simulink model "FreqAdaptive"  (R2018a)
settings: Solver=ode8  StartTime=0.0  StopTime=Ttot  FixedStep=Ts  RelTol=1e-3
values from neighbouring files (symbols this model uses):
  Fn = 60    [Equivalency_Script.m]    (also in FreqAdaptiveFFT_Script.m; FreqAdaptive_Script.m; ShortPulse_Script.m)
  Ts = Ts_control / 60    (= 9.25925925926e-07)    [Equivalency_Script.m]    (also in FreqAdaptiveFFT_Script.m; FreqAdaptive_Script.m; ShortPulse_Script.m)
  Ts_control = 1/(300*Fn)    (= 5.55555555556e-05)    [Equivalency_Script.m]    (also in FreqAdaptiveFFT_Script.m; FreqAdaptive_Script.m; ShortPulse_Script.m)
libraries: powerlib x3, DSCdq_Library x2, powerlib_meascontrol x2
settings Model: SimulationMode=accelerator  Creator=daniemot  LastModifiedBy=daniemot
settings SolverCC: AutoInsertRateTranBlk=on
settings DataIOCC: ExternalInput=getinputstruct(WN_50mF_op_snapshot1)  InitialState=getstatestruct(WN_50mF_op_snapshot1)  SaveFinalState=on  SaveFormat=StructureWithTime  SaveOutput=off  SignalLogging=off  DSMLogging=off  SaveTime=off
settings DebuggingCC: ReadBeforeWriteMsg=DisableAll  WriteAfterWriteMsg=DisableAll  WriteAfterReadMsg=DisableAll  MultiTaskDSMMsg=none  UnconnectedInputMsg=none  UnconnectedOutputMsg=none  UnconnectedLineMsg=none
settings ModelReferenceCC: UpdateModelReferenceTargets=IfOutOfDate
settings SFSimCC: SFSimEcho=off

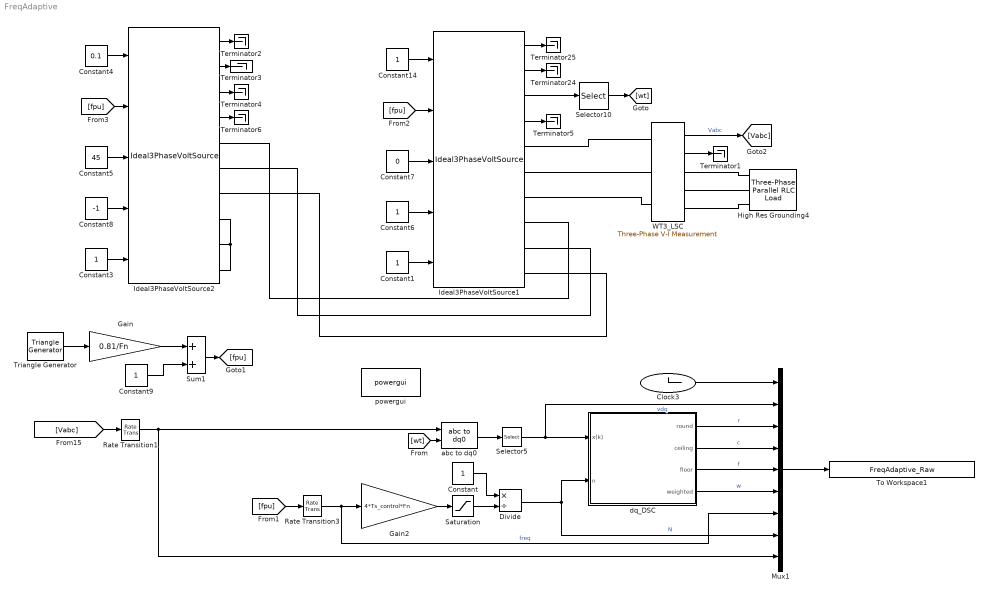
== system FreqAdaptive ==
  Clock3 : Clock
  Constant{,1,3,6,9,14} (6 alike) : Constant
  Constant4 : Constant  Value=0.1
  Constant5 : Constant  Value=45
  Constant7 : Constant  Value=0
  Constant8 : Constant  Value=-1
  Divide : Product  Inputs=*/
  Gain : Gain  Gain=0.81/Fn
  Gain2 : Gain  Gain=4*Ts_control*Fn
  High Res Grounding4 : powerlib/Elements/Three-Phase Parallel RLC Load  LConnTagsString=A|B|C  Configuration=Y (grounded)  NominalVoltage=(1/2^0.5)*3^0.5  Vabc=[1e3 1e3 1e3]  Vabcp=[1e3 1e3 1e3]  NominalFrequency=Fn  UnbalancedPower=off  ActivePower=3/2  InductivePower=0  CapacitivePower=0  Pabc=[10e3 9e3 11e3]  QLabc=[100 90 110]  QCabc=[100 90 110]  Pabcp=[10e3 9e3 11e3]  QLabcp=[100 90 110]  QCabcp=[100 90 110]  Measurements=None  LoadType=constant Z
  Ideal3PhaseVoltSource1 : DSCdq_Library/Ideal3PhaseVoltSource  BaseAmp=1  fn=Fn
  Ideal3PhaseVoltSource2 : DSCdq_Library/Ideal3PhaseVoltSource  BaseAmp=1  fn=Fn
  Mux1 : Mux  Inputs=9
  Rate Transition1 : RateTransition  OutPortSampleTime=Ts_control
  Rate Transition3 : RateTransition  InitialCondition=1  OutPortSampleTime=Ts_control
  Saturation : Saturate  UpperLimit=inf  LowerLimit=0.000001
  Selector10 : Selector  InputPortWidth=3  IndexOptions=Index vector (dialog)  Indices=[1]  OutputSizes=1
  Selector5 : Selector  InputPortWidth=3  IndexOptions=Index vector (dialog)  Indices=[1 2]  OutputSizes=1
  Sum1 : Sum
  Terminator{1..6,24..25} (8 alike) : Terminator
  To Workspace1 : ToWorkspace  VariableName=FreqAdaptive_Raw  SampleTime=Ts_control
      settings: Save2DSignal=2-D array (concatenate along first dimension)
  Triangle Generator : powerlib_meascontrol/Pulse & Signal Generators/Triangle Generator  Freq=2  Phase=90  Ts=0
  WT3_LSC : powerlib/Measurements/Three-Phase V-I Measurement  VoltageMeasurement=phase-to-ground  SetLabelV=off  LabelV=vgrid  Vpu=off  VpuLL=off  CurrentMeasurement=yes  SetLabelI=off  LabelI=igrid  Ipu=off  Pbase=sn  Vbase=uab  OutputType=Complex  PhasorSimulation=off  PSBequivalent=0
  abc to dq0 : powerlib_meascontrol/Transformations/abc to dq0  Alignment=90 degrees behind phase A axis
  dq_DSC : Subsystem  TreatAsAtomicUnit=on  SystemSampleTime=Ts  mask{Ts=Ts_control, nmax=200}
      mask prompts: Ts "Sample times [s]"; nmax "Maximum delay nmax:"
      mask Display: fprintf('y(k)=0.5(x(k)+x(k-n))');
  powergui : powerlib/powergui  Priority=1  SimulationMode=Discrete  SampleTime=Ts  frequency=60  Iterations=50  frequencyindice=0  Pbase=100e6  ErrMax=1e-4  UnitsV=kV  UnitsW=MW  buscounter=0  FunctionMessages=off  echomessages=off  EnableUseOfTLC=off  CurrentSourceSwitches=off  DisableSnubberDevices=off  DisableRonSwitches=off  DisableVfSwitches=off  DisplayEquations=off  SolverType=Tustin/Backward Euler (TBE)  Interpol=off  ExternalGateDelay=off  methode=off  Ts=100  x0status=blocks  SPID=off  SwTol=0  HookPort=off  RestoreLinks=warning  ResistiveCurrentMeasurement=off  Frange=[60:1:1600]  Ylog=on  Xlog=on  ShowGrid=on  save=off  variable=ZData  structure=0  ZoomFFT=off  StartTime=0.0  cycles=1  DisplayStyle=1  fundamental=60  FreqAxis=off  MaxFrequency=1000  frequencyindicesteady=1  RmsSteady=1  display=off
  wires:
  Constant6/1 -> Ideal3PhaseVoltSource1/4
  Constant7/1 -> Ideal3PhaseVoltSource1/3
  Triangle Generator/1 -> Gain/1
  Ideal3PhaseVoltSource1/3 -> Selector10/1
  Ideal3PhaseVoltSource1/2 -> Terminator24/1
  Ideal3PhaseVoltSource1/1 -> Terminator25/1
  WT3_LSC/1 -> [Vabc]  "Vabc"
  Ideal3PhaseVoltSource1/4 -> Terminator5/1
  Clock3/1 -> Mux1/1
  Mux1/1 -> To Workspace1/1
  Constant14/1 -> Ideal3PhaseVoltSource1/1
  Constant1/1 -> Ideal3PhaseVoltSource1/5
  WT3_LSC/2 -> Terminator1/1
  Selector5/1 -> Mux1/2, dq_DSC/1(x(k))  "vdq"
  [wt] -> abc to dq0/2
  abc to dq0/1 -> Selector5/1
  [Vabc] -> Rate Transition1/1
  Divide/1 -> Mux1/8, dq_DSC/2(n)  "N"
  Constant/1 -> Divide/1
  [fpu] -> Rate Transition3/1
  Gain2/1 -> Saturation/1
  Saturation/1 -> Divide/2
  dq_DSC/1(round) -> Mux1/3  "r"
  dq_DSC/2(ceiling) -> Mux1/4  "c"
  dq_DSC/3(floor) -> Mux1/5  "f"
  dq_DSC/4(weighted) -> Mux1/6  "w"
  Rate Transition3/1 -> Mux1/7, Gain2/1  "freq"
  Ideal3PhaseVoltSource2/1 -> Terminator2/1
  Ideal3PhaseVoltSource2/2 -> Terminator3/1
  Ideal3PhaseVoltSource2/3 -> Terminator4/1
  Ideal3PhaseVoltSource2/4 -> Terminator6/1
  Constant3/1 -> Ideal3PhaseVoltSource2/5
  [fpu] -> Ideal3PhaseVoltSource2/2
  Constant4/1 -> Ideal3PhaseVoltSource2/1
  Constant5/1 -> Ideal3PhaseVoltSource2/3
  Constant8/1 -> Ideal3PhaseVoltSource2/4
  Sum1/1 -> [fpu]
  Gain/1 -> Sum1/1
  Constant9/1 -> Sum1/2
  Rate Transition1/1 -> abc to dq0/1, Mux1/9
  [fpu] -> Ideal3PhaseVoltSource1/2
  Selector10/1 -> [wt]
  connections:
  Ideal3PhaseVoltSource1/RConn1 -- WT3_LSC/LConn1
  Ideal3PhaseVoltSource1/RConn3 -- WT3_LSC/LConn3
  Ideal3PhaseVoltSource1/RConn2 -- WT3_LSC/LConn2
  High Res Grounding4/LConn1 -- WT3_LSC/RConn1
  High Res Grounding4/LConn2 -- WT3_LSC/RConn2
  High Res Grounding4/LConn3 -- WT3_LSC/RConn3
  Ideal3PhaseVoltSource2/RConn4 -- Ideal3PhaseVoltSource2/RConn6 -- Ideal3PhaseVoltSource2/RConn5
  Ideal3PhaseVoltSource1/RConn6 -- Ideal3PhaseVoltSource2/RConn3
  Ideal3PhaseVoltSource1/RConn5 -- Ideal3PhaseVoltSource2/RConn2
  Ideal3PhaseVoltSource1/RConn4 -- Ideal3PhaseVoltSource2/RConn1

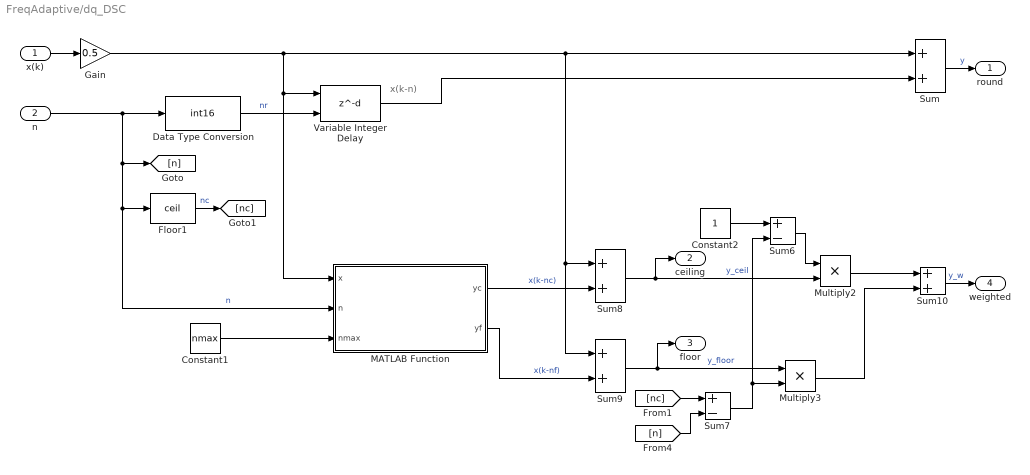
== system FreqAdaptive/dq_DSC ==
  note: x(k-n)
  x(k) : Inport
  n : Inport  Port=2
  Constant1 : Constant  Value=nmax
  Constant2 : Constant
  Data Type Conversion : DataTypeConversion  OutDataTypeStr=int16  RndMeth=Round  SaturateOnIntegerOverflow=on
  Floor1 : Rounding  Operator=ceil
  Gain : Gain  Gain=0.5
  MATLAB Function : MATLAB Function  TreatAsAtomicUnit=on  SystemSampleTime=Ts_control
  Multiply2 : Product
  Multiply3 : Product
  Sum{,8..10} (4 alike) : Sum
  Sum6 : Sum  Inputs=+-
  Sum7 : Sum  Inputs=+-
  Variable Integer Delay : Delay  DelayLengthSource=Input port  DelayLength=200  DelayLengthUpperLimit=nmax  SampleTime=Ts
      settings: InputPortMap=u0,p1
  round : Outport
  ceiling : Outport  Port=2
  floor : Outport  Port=3
  weighted : Outport  Port=4
  wires:
  Sum/1 -> round/1  "y"
  Data Type Conversion/1 -> Variable Integer Delay/2  "nr"
  Floor1/1 -> [nc]  "nc"
  Variable Integer Delay/1 -> Sum/2
  x(k)/1 -> Gain/1
  n/1 -> Data Type Conversion/1, Floor1/1, MATLAB Function/2(n), [n]  "n"
  Constant1/1 -> MATLAB Function/3(nmax)
  [n] -> Sum7/2
  MATLAB Function/1(yc) -> Sum8/2  "x(k-nc)"
  Sum7/1 -> Sum6/2, Multiply3/2
  Constant2/1 -> Sum6/1
  Sum6/1 -> Multiply2/1
  MATLAB Function/2(yf) -> Sum9/2  "x(k-nf)"
  Sum8/1 -> ceiling/1, Multiply2/2  "y_ceil"
  Sum9/1 -> floor/1, Multiply3/1  "y_floor"
  Sum10/1 -> weighted/1  "y_w"
  Gain/1 -> Sum/1, Sum9/1, Sum8/1, Variable Integer Delay/1, MATLAB Function/1(x)
  Multiply3/1 -> Sum10/2
  [nc] -> Sum7/1
  Multiply2/1 -> Sum10/1

== matlab function FreqAdaptive/dq_DSC/MATLAB Function ==
  data: x input; yc output; n input; yf output; nmax input
function [yc,    yf]  = CircBuff_Delay_CeilFloor(x, n, nmax)
%% %%%%%%%%%%%%%%%%%%%%%%%%%%%%%%%%%%%%%%%%%%%%%%%%%%%%%%%%%%%%%%%%%%%%%%%%
% Circular Buffer 
% By: Mota
% Revision history:
%       2021-07-16: first release
%
%%Interface  
%   Inputs
%       x : must be a vector pf two values
%       n : delay in samples (float, ideal delay is time was continuous)
%       nmax : max size of circular buffer, ONLY used in FIRST CYCLE
%
%   Output
%       yc = x(k - ceil(n))
%       yf = x(k - floor(n))
% 

persistent CB       % circular buffer, created with zeros in first cycle
persistent ins_p    % insertion pointer, integer, zero -> Nmax-1
persistent Nmax     % Buffer lenght, updated ONLY in FIRST CYCLE


%% Initialization of persistent variables
if isempty(Nmax)
    if nmax < 5     % Hardcoded minimum lenght of buffer (arbitrary)
        Nmax = 5;
    else 
        Nmax = round(nmax); % No limit for maximum lenght of buffer 
    end
    
    CB = zeros(Nmax, 2);    % circular buffer
                            % Nmax lines x 2 columns 
                            % Column 1: ceiling 
                            % Column 2: floor
    
    ins_p = 0;      % Insertion pointer initialization
    
end

%% %%%%%%%%%%%%%%%%%%%%%%%%%%%%%%%%%%%%%%%%%%%%%%%%%%%%%%%%%%%%%%%%%%%%%%
% Insertion of current values
%%%%%%%%%%%%%%%%%%%%%%%%%%%%%%%%%%%%%%%%%%%%%%%%%%%%%%%%%%%%%%%%%%%%%%%%%
CB(ins_p + 1, 1) = x(1);    
CB(ins_p + 1, 2) = x(2);

%% %%%%%%%%%%%%%%%%%%%%%%%%%%%%%%%%%%%%%%%%%%%%%%%%%%%%%%%%%%%%%%%%%%%%%%
% Retrieval pointer calculation
%   Be careful with confusion of indices
%       Matlab index for array:     1, 2,... Nmax
%       Insertion pointer values:   0, 1,... Nmax - 1
%%%%%%%%%%%%%%%%%%%%%%%%%%%%%%%%%%%%%%%%%%%%%%%%%%%%%%%%%%%%%%%%%%%%%%%%%
if n >= 1       
    if n <= Nmax - 1    % if 1 >= n >= Nmax - 1 
                        % n cannot be equal to Nmax, or else the retrieval
                        % pointers retreat back to the the insertion
                        % pointer.
                                
        p_r_c = mod(ins_p - ceil(n), Nmax); % ceiling retrieval pointer
        p_r_f = mod(ins_p - floor(n), Nmax); % floor retrieval pointer
    
    else
        % The maximum delay is Nmax - 1
        p_r_c = mod(ins_p - Nmax - 1, Nmax);
        p_r_f = mod(ins_p - Nmax - 1, Nmax);
    end
else
    % Minimul delay is zero
    p_r_c = ins_p;
    p_r_f = ins_p;
end
    
%% %%%%%%%%%%%%%%%%%%%%%%%%%%%%%%%%%%%%%%%%%%%%%%%%%%%%%%%%%%%%%%%%%%%%%%
% Temporary variables with retrieved values
%   CB indexes: 1, 2, ... Nmax
%%%%%%%%%%%%%%%%%%%%%%%%%%%%%%%%%%%%%%%%%%%%%%%%%%%%%%%%%%%%%%%%%%%%%%%%%
col1_c = CB(p_r_c + 1, 1); 
col1_f = CB(p_r_f + 1, 1);

col2_c = CB(p_r_c + 1, 2);
col2_f = CB(p_r_f + 1, 2);

%% %%%%%%%%%%%%%%%%%%%%%%%%%%%%%%%%%%%%%%%%%%%%%%%%%%%%%%%%%%%%%%%%%%%%%%
% Outputs vectors
%%%%%%%%%%%%%%%%%%%%%%%%%%%%%%%%%%%%%%%%%%%%%%%%%%%%%%%%%%%%%%%%%%%%%%%%%
yc = [col1_c col2_c];
yf = [col1_f col2_f];

%% %%%%%%%%%%%%%%%%%%%%%%%%%%%%%%%%%%%%%%%%%%%%%%%%%%%%%%%%%%%%%%%%%%%%%%
% Update Outputs vectors
%%%%%%%%%%%%%%%%%%%%%%%%%%%%%%%%%%%%%%%%%%%%%%%%%%%%%%%%%%%%%%%%%%%%%%%%%
ins_p = mod(ins_p + 1, Nmax);
